simulink model "Lab1_parameter_estimation_student"  (R2024b)
settings: Solver=FixedStepAuto  StartTime=0.0  StopTime=inf  FixedStep=0.001  RelTol=1e-3
undefined symbols (not defined in the file): motor_B, motor_Eff, motor_J, motor_Ke, motor_L, motor_R
libraries: simulink x1
settings Model: Creator=tanawatp  LastModifiedBy=acer
settings RTWCC: GPUComputeCapability=3.5

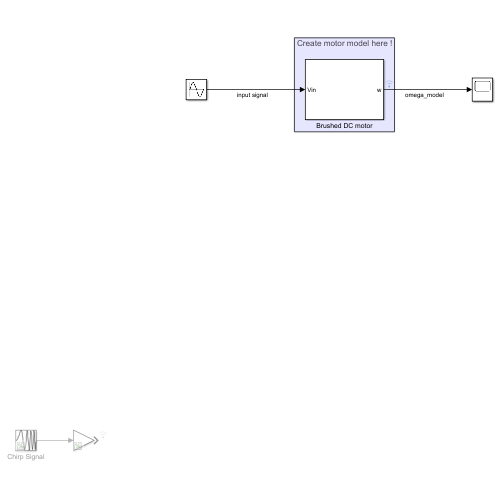
[thumbnail: Simulink's stored preview of the top-level diagram]
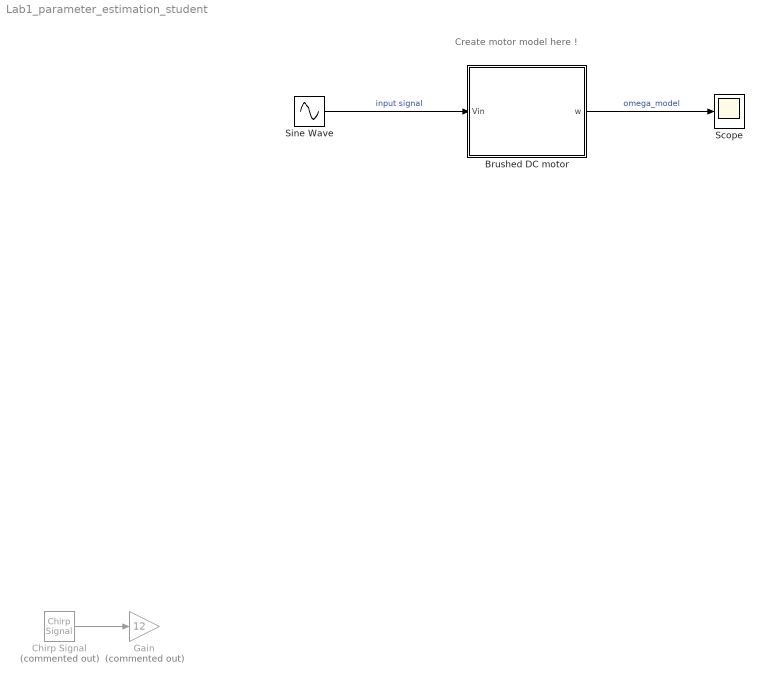
== system Lab1_parameter_estimation_student ==
  note: Create motor model here !
  Brushed DC motor : Subsystem
  Chirp Signal : simulink/Sources/Chirp Signal  Commented=on  f1=0.1  T=40  f2=5
  Gain : Gain  Commented=on  Gain=12
  Scope : Scope
  Sine Wave : Sin  Amplitude=12  Frequency=2*pi * 0.1  SampleTime=0
  wires:
  Brushed DC motor/1(w) -> Scope/1  "omega_model"
  Chirp Signal/1 -> Gain/1
  Sine Wave/1 -> Brushed DC motor/1(Vin)  "input signal"

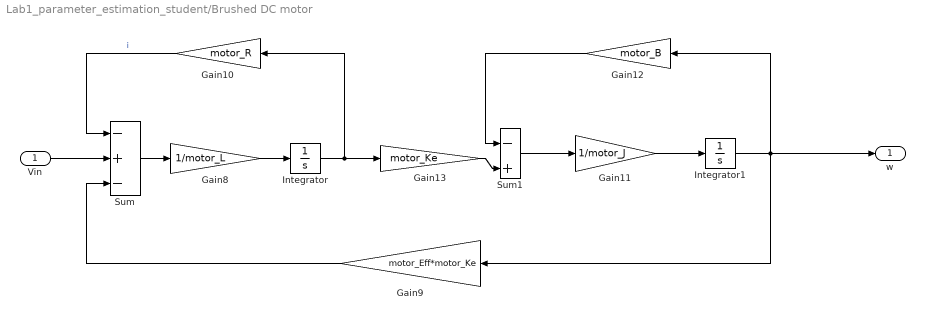
== system Lab1_parameter_estimation_student/Brushed DC motor ==
  Vin : Inport
  Gain10 : Gain  Gain=motor_R
  Gain11 : Gain  Gain=1/motor_J
  Gain12 : Gain  Gain=motor_B
  Gain13 : Gain  Gain=motor_Ke
  Gain8 : Gain  Gain=1/motor_L
  Gain9 : Gain  Gain=motor_Eff*motor_Ke
  Integrator : Integrator
  Integrator1 : Integrator
  Sum : Sum  Inputs=-+-
  Sum1 : Sum  Inputs=-|+|
  w : Outport
  wires:
  Vin/1 -> Sum/2
  Sum/1 -> Gain8/1
  Gain8/1 -> Integrator/1
  Integrator/1 -> Gain13/1, Gain10/1
  Gain10/1 -> Sum/1  "i"
  Gain13/1 -> Sum1/2
  Sum1/1 -> Gain11/1
  Integrator1/1 -> Gain9/1, Gain12/1, w/1
  Gain12/1 -> Sum1/1
  Gain11/1 -> Integrator1/1
  Gain9/1 -> Sum/3
